simulink model "REGULATORS"  (R2017b)
settings: Solver=VariableStepAuto  StartTime=0.0  StopTime=500  RelTol=1e-3
values from neighbouring files (symbols this model uses):
  A = [dh1dh1 dh1dh2; dh2dh1 dh2dh2]    [SSV_milan.m]    (also in identifikace.m = -0.066; linear_systim.m)
  a_con = 0.075    [SSV_milan.m]
  B = [ dh1du dh1dvt dh1dvo; dh2du dh2dvt dh2dvo ]    [SSV_milan.m]    (also in identifikace.m = -0.0144; linear_systim.m)
  b_con = 0.013    [SSV_milan.m]
  C = [1 0; 0 1]    [SSV_milan.m]    (also in identifikace.m = -0.02; linear_systim.m)
  c_con = 0.02    [SSV_milan.m]
  D = [ 0 0 0; 0 0 0]    [SSV_milan.m]    (also in linear_systim.m)
  d_con = 2.4    [SSV_milan.m]
  h10 = 0.18    [SSV_milan.m]    (also in identifikace_parametru.m = 0.066; linear_systim.m = 0.16)
  h1off = 0.045    [SSV_milan.m]    (also in linear_systim.m = 0.05)
  h20 = 0.08    [SSV_milan.m]    (also in identifikace_parametru.m = 0.175; linear_systim.m = 0.14)
  u0 = 0.4    [SSV_milan.m]    (also in linear_systim.m)
  vO = 1    [SSV_milan.m]    (also in linear_systim.m = 0)
  vT = 1    [SSV_milan.m]    (also in linear_systim.m = 0.5)
libraries: simulink x6
settings Model: Creator=ladislav  LastModifiedBy=ladislav

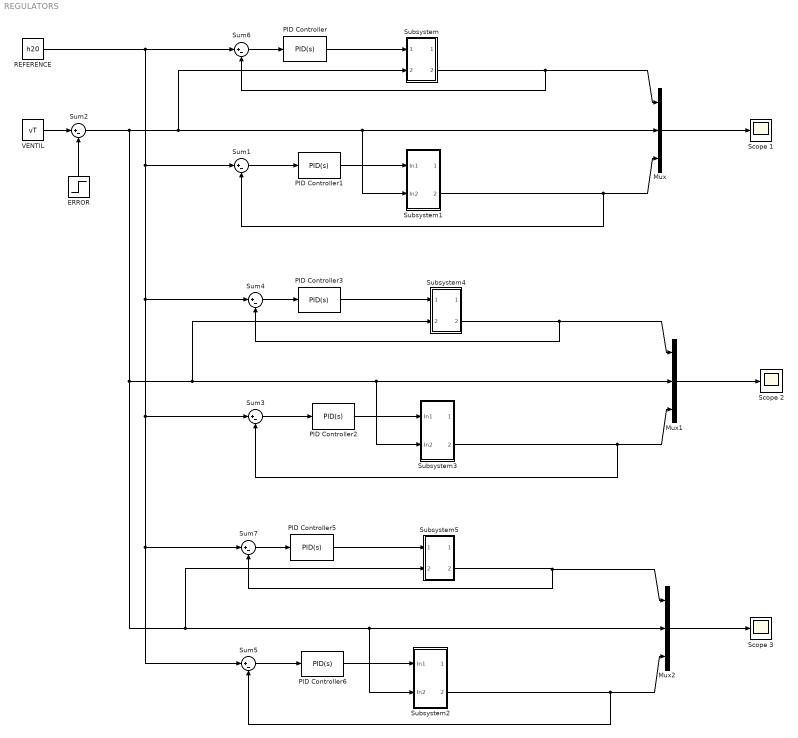
== system REGULATORS ==
  ERROR : Step  Time=200  After=0.2  SampleTime=0  ZeroCross=off
  Mux : Mux  Inputs=3
  Mux1 : Mux  Inputs=3
  Mux2 : Mux  Inputs=3
  PID Controller : simulink/Continuous/PID Controller  Controller=PID  TimeDomain=Continuous-time  SampleTime=-1  IntegratorMethod=Forward Euler  FilterMethod=Forward Euler  Form=Parallel  UseFilter=on  ControllerParametersSource=internal  P=4.4816  I=0.2801  D=0  N=100  InitialConditionSource=internal  InitialConditionForIntegrator=0  InitialConditionForFilter=0  ExternalReset=none  LimitOutput=on  UpperSaturationLimit=1  LowerSaturationLimit=0  LinearizeAsGain=on  AntiWindupMode=none  Kb=1  TrackingMode=off  Kt=1  PParamMin=[]  PParamMax=[]  IParamMin=[]  IParamMax=[]  DParamMin=[]  DParamMax=[]  NParamMin=[]  NParamMax=[]  KbParamMin=[]  KbParamMax=[]  KtParamMin=[]  KtParamMax=[]  POutMin=[]  POutMax=[]  IOutMin=[]  IOutMax=[]  DOutMin=[]  DOutMax=[]  NOutMin=[]  NOutMax=[]  KbOutMin=[]  KbOutMax=[]  KtOutMin=[]  KtOutMax=[]  IntegratorOutMin=[]  IntegratorOutMax=[]  FilterOutMin=[]  FilterOutMax=[]  SumOutMin=[]  SumOutMax=[]  SumI1OutMin=[]  SumI1OutMax=[]  SumI2OutMin=[]  SumI2OutMax=[]  SumI3OutMin=[]  SumI3OutMax=[]  SumDOutMin=[]  SumDOutMax=[]  SaturationOutMin=[]  SaturationOutMax=[]  IntegratorContinuousStateAttributes=''  IntegratorStateMustResolveToSignalObject=off  IntegratorRTWStateStorageClass=Auto  FilterContinuousStateAttributes=''  FilterStateMustResolveToSignalObject=off  FilterRTWStateStorageClass=Auto  DifferentiatorICPrevScaledInput=0  DifferentiatorOutMin=[]  DifferentiatorOutMax=[]  InitialConditionSetting=State (most efficient)  FilterDiffOutCoefMin=[]  FilterDiffOutCoefMax=[]  SumDenOutMin=[]  SumDenOutMax=[]  SumNumOutMin=[]  SumNumOutMax=[]  ReciprocalOutMin=[]  ReciprocalOutMax=[]  DivideOutMin=[]  DivideOutMax=[]  TunerSelectOption=Transfer Function Based (PID Tuner App)
  PID Controller1 : simulink/Continuous/PID Controller  Controller=PID  TimeDomain=Continuous-time  SampleTime=-1  IntegratorMethod=Forward Euler  FilterMethod=Forward Euler  Form=Parallel  UseFilter=on  ControllerParametersSource=internal  P=4.4816  I=0.2801  D=0  N=100  InitialConditionSource=internal  InitialConditionForIntegrator=0  InitialConditionForFilter=0  ExternalReset=none  LimitOutput=on  UpperSaturationLimit=1.0  LowerSaturationLimit=0  LinearizeAsGain=on  AntiWindupMode=none  Kb=1  TrackingMode=off  Kt=1  PParamMin=[]  PParamMax=[]  IParamMin=[]  IParamMax=[]  DParamMin=[]  DParamMax=[]  NParamMin=[]  NParamMax=[]  KbParamMin=[]  KbParamMax=[]  KtParamMin=[]  KtParamMax=[]  POutMin=[]  POutMax=[]  IOutMin=[]  IOutMax=[]  DOutMin=[]  DOutMax=[]  NOutMin=[]  NOutMax=[]  KbOutMin=[]  KbOutMax=[]  KtOutMin=[]  KtOutMax=[]  IntegratorOutMin=[]  IntegratorOutMax=[]  FilterOutMin=[]  FilterOutMax=[]  SumOutMin=[]  SumOutMax=[]  SumI1OutMin=[]  SumI1OutMax=[]  SumI2OutMin=[]  SumI2OutMax=[]  SumI3OutMin=[]  SumI3OutMax=[]  SumDOutMin=[]  SumDOutMax=[]  SaturationOutMin=[]  SaturationOutMax=[]  IntegratorContinuousStateAttributes=''  IntegratorStateMustResolveToSignalObject=off  IntegratorRTWStateStorageClass=Auto  FilterContinuousStateAttributes=''  FilterStateMustResolveToSignalObject=off  FilterRTWStateStorageClass=Auto  DifferentiatorICPrevScaledInput=0  DifferentiatorOutMin=[]  DifferentiatorOutMax=[]  InitialConditionSetting=State (most efficient)  FilterDiffOutCoefMin=[]  FilterDiffOutCoefMax=[]  SumDenOutMin=[]  SumDenOutMax=[]  SumNumOutMin=[]  SumNumOutMax=[]  ReciprocalOutMin=[]  ReciprocalOutMax=[]  DivideOutMin=[]  DivideOutMax=[]  TunerSelectOption=Transfer Function Based (PID Tuner App)
  PID Controller2 : simulink/Continuous/PID Controller  Controller=PID  TimeDomain=Continuous-time  SampleTime=-1  IntegratorMethod=Forward Euler  FilterMethod=Forward Euler  Form=Parallel  UseFilter=on  ControllerParametersSource=internal  P=37.28  I=5.78  D=1.447  N=100  InitialConditionSource=internal  InitialConditionForIntegrator=0  InitialConditionForFilter=0  ExternalReset=none  LimitOutput=on  UpperSaturationLimit=1  LowerSaturationLimit=0  LinearizeAsGain=on  AntiWindupMode=none  Kb=1  TrackingMode=off  Kt=1  PParamMin=[]  PParamMax=[]  IParamMin=[]  IParamMax=[]  DParamMin=[]  DParamMax=[]  NParamMin=[]  NParamMax=[]  KbParamMin=[]  KbParamMax=[]  KtParamMin=[]  KtParamMax=[]  POutMin=[]  POutMax=[]  IOutMin=[]  IOutMax=[]  DOutMin=[]  DOutMax=[]  NOutMin=[]  NOutMax=[]  KbOutMin=[]  KbOutMax=[]  KtOutMin=[]  KtOutMax=[]  IntegratorOutMin=[]  IntegratorOutMax=[]  FilterOutMin=[]  FilterOutMax=[]  SumOutMin=[]  SumOutMax=[]  SumI1OutMin=[]  SumI1OutMax=[]  SumI2OutMin=[]  SumI2OutMax=[]  SumI3OutMin=[]  SumI3OutMax=[]  SumDOutMin=[]  SumDOutMax=[]  SaturationOutMin=[]  SaturationOutMax=[]  IntegratorContinuousStateAttributes=''  IntegratorStateMustResolveToSignalObject=off  IntegratorRTWStateStorageClass=Auto  FilterContinuousStateAttributes=''  FilterStateMustResolveToSignalObject=off  FilterRTWStateStorageClass=Auto  DifferentiatorICPrevScaledInput=0  DifferentiatorOutMin=[]  DifferentiatorOutMax=[]  InitialConditionSetting=State (most efficient)  FilterDiffOutCoefMin=[]  FilterDiffOutCoefMax=[]  SumDenOutMin=[]  SumDenOutMax=[]  SumNumOutMin=[]  SumNumOutMax=[]  ReciprocalOutMin=[]  ReciprocalOutMax=[]  DivideOutMin=[]  DivideOutMax=[]  TunerSelectOption=Transfer Function Based (PID Tuner App)
  PID Controller3 : simulink/Continuous/PID Controller  Controller=PID  TimeDomain=Continuous-time  SampleTime=-1  IntegratorMethod=Forward Euler  FilterMethod=Forward Euler  Form=Parallel  UseFilter=on  ControllerParametersSource=internal  P=37.28  I=5.78  D=1.447  N=100  InitialConditionSource=internal  InitialConditionForIntegrator=0  InitialConditionForFilter=0  ExternalReset=none  LimitOutput=on  UpperSaturationLimit=1  LowerSaturationLimit=0  LinearizeAsGain=on  AntiWindupMode=none  Kb=1  TrackingMode=off  Kt=1  PParamMin=[]  PParamMax=[]  IParamMin=[]  IParamMax=[]  DParamMin=[]  DParamMax=[]  NParamMin=[]  NParamMax=[]  KbParamMin=[]  KbParamMax=[]  KtParamMin=[]  KtParamMax=[]  POutMin=[]  POutMax=[]  IOutMin=[]  IOutMax=[]  DOutMin=[]  DOutMax=[]  NOutMin=[]  NOutMax=[]  KbOutMin=[]  KbOutMax=[]  KtOutMin=[]  KtOutMax=[]  IntegratorOutMin=[]  IntegratorOutMax=[]  FilterOutMin=[]  FilterOutMax=[]  SumOutMin=[]  SumOutMax=[]  SumI1OutMin=[]  SumI1OutMax=[]  SumI2OutMin=[]  SumI2OutMax=[]  SumI3OutMin=[]  SumI3OutMax=[]  SumDOutMin=[]  SumDOutMax=[]  SaturationOutMin=[]  SaturationOutMax=[]  IntegratorContinuousStateAttributes=''  IntegratorStateMustResolveToSignalObject=off  IntegratorRTWStateStorageClass=Auto  FilterContinuousStateAttributes=''  FilterStateMustResolveToSignalObject=off  FilterRTWStateStorageClass=Auto  DifferentiatorICPrevScaledInput=0  DifferentiatorOutMin=[]  DifferentiatorOutMax=[]  InitialConditionSetting=State (most efficient)  FilterDiffOutCoefMin=[]  FilterDiffOutCoefMax=[]  SumDenOutMin=[]  SumDenOutMax=[]  SumNumOutMin=[]  SumNumOutMax=[]  ReciprocalOutMin=[]  ReciprocalOutMax=[]  DivideOutMin=[]  DivideOutMax=[]  TunerSelectOption=Transfer Function Based (PID Tuner App)
  PID Controller5 : simulink/Continuous/PID Controller  Controller=PID  TimeDomain=Continuous-time  SampleTime=-1  IntegratorMethod=Forward Euler  FilterMethod=Forward Euler  Form=Parallel  UseFilter=on  ControllerParametersSource=internal  P=43.1  I=0  D=86.2  N=100  InitialConditionSource=internal  InitialConditionForIntegrator=0  InitialConditionForFilter=0  ExternalReset=none  LimitOutput=on  UpperSaturationLimit=1  LowerSaturationLimit=0  LinearizeAsGain=on  AntiWindupMode=none  Kb=1  TrackingMode=off  Kt=1  PParamMin=[]  PParamMax=[]  IParamMin=[]  IParamMax=[]  DParamMin=[]  DParamMax=[]  NParamMin=[]  NParamMax=[]  KbParamMin=[]  KbParamMax=[]  KtParamMin=[]  KtParamMax=[]  POutMin=[]  POutMax=[]  IOutMin=[]  IOutMax=[]  DOutMin=[]  DOutMax=[]  NOutMin=[]  NOutMax=[]  KbOutMin=[]  KbOutMax=[]  KtOutMin=[]  KtOutMax=[]  IntegratorOutMin=[]  IntegratorOutMax=[]  FilterOutMin=[]  FilterOutMax=[]  SumOutMin=[]  SumOutMax=[]  SumI1OutMin=[]  SumI1OutMax=[]  SumI2OutMin=[]  SumI2OutMax=[]  SumI3OutMin=[]  SumI3OutMax=[]  SumDOutMin=[]  SumDOutMax=[]  SaturationOutMin=[]  SaturationOutMax=[]  IntegratorContinuousStateAttributes=''  IntegratorStateMustResolveToSignalObject=off  IntegratorRTWStateStorageClass=Auto  FilterContinuousStateAttributes=''  FilterStateMustResolveToSignalObject=off  FilterRTWStateStorageClass=Auto  DifferentiatorICPrevScaledInput=0  DifferentiatorOutMin=[]  DifferentiatorOutMax=[]  InitialConditionSetting=State (most efficient)  FilterDiffOutCoefMin=[]  FilterDiffOutCoefMax=[]  SumDenOutMin=[]  SumDenOutMax=[]  SumNumOutMin=[]  SumNumOutMax=[]  ReciprocalOutMin=[]  ReciprocalOutMax=[]  DivideOutMin=[]  DivideOutMax=[]  TunerSelectOption=Transfer Function Based (PID Tuner App)
  PID Controller6 : simulink/Continuous/PID Controller  Controller=PID  TimeDomain=Continuous-time  SampleTime=-1  IntegratorMethod=Forward Euler  FilterMethod=Forward Euler  Form=Parallel  UseFilter=on  ControllerParametersSource=internal  P=43.1  I=0  D=86.2  N=100  InitialConditionSource=internal  InitialConditionForIntegrator=0  InitialConditionForFilter=0  ExternalReset=none  LimitOutput=on  UpperSaturationLimit=1  LowerSaturationLimit=0  LinearizeAsGain=on  AntiWindupMode=none  Kb=1  TrackingMode=off  Kt=1  PParamMin=[]  PParamMax=[]  IParamMin=[]  IParamMax=[]  DParamMin=[]  DParamMax=[]  NParamMin=[]  NParamMax=[]  KbParamMin=[]  KbParamMax=[]  KtParamMin=[]  KtParamMax=[]  POutMin=[]  POutMax=[]  IOutMin=[]  IOutMax=[]  DOutMin=[]  DOutMax=[]  NOutMin=[]  NOutMax=[]  KbOutMin=[]  KbOutMax=[]  KtOutMin=[]  KtOutMax=[]  IntegratorOutMin=[]  IntegratorOutMax=[]  FilterOutMin=[]  FilterOutMax=[]  SumOutMin=[]  SumOutMax=[]  SumI1OutMin=[]  SumI1OutMax=[]  SumI2OutMin=[]  SumI2OutMax=[]  SumI3OutMin=[]  SumI3OutMax=[]  SumDOutMin=[]  SumDOutMax=[]  SaturationOutMin=[]  SaturationOutMax=[]  IntegratorContinuousStateAttributes=''  IntegratorStateMustResolveToSignalObject=off  IntegratorRTWStateStorageClass=Auto  FilterContinuousStateAttributes=''  FilterStateMustResolveToSignalObject=off  FilterRTWStateStorageClass=Auto  DifferentiatorICPrevScaledInput=0  DifferentiatorOutMin=[]  DifferentiatorOutMax=[]  InitialConditionSetting=State (most efficient)  FilterDiffOutCoefMin=[]  FilterDiffOutCoefMax=[]  SumDenOutMin=[]  SumDenOutMax=[]  SumNumOutMin=[]  SumNumOutMax=[]  ReciprocalOutMin=[]  ReciprocalOutMax=[]  DivideOutMin=[]  DivideOutMax=[]  TunerSelectOption=Transfer Function Based (PID Tuner App)
  REFERENCE : Constant  Value=h20
  Scope 1 : Scope
  Scope 2 : Scope
  Scope 3 : Scope
  Subsystem : Subsystem
  Subsystem1 : Subsystem
  Subsystem2 : Subsystem
  Subsystem3 : Subsystem
  Subsystem4 : Subsystem
  Subsystem5 : Subsystem
  Sum{1..7} (7 alike) : Sum  Inputs=|+-
  "VENTIL " : Constant  Value=vT
  wires:
  Sum6/1 -> PID Controller/1
  Subsystem/2(Out2) -> Mux/1, Sum6/2
  PID Controller/1 -> Subsystem/1(In1)
  Sum1/1 -> PID Controller1/1
  PID Controller1/1 -> Subsystem1/1(In1)
  Subsystem1/2(Out2) -> Mux/3, Sum1/2
  Mux/1 -> Scope 1/1
  "VENTIL "/1 -> Sum2/1
  ERROR/1 -> Sum2/2
  PID Controller3/1 -> Subsystem4/1(In1)
  Sum3/1 -> PID Controller2/1
  PID Controller2/1 -> Subsystem3/1(In1)
  Sum4/1 -> PID Controller3/1
  Subsystem3/2(Out2) -> Mux1/3, Sum3/2
  Subsystem4/2(Out2) -> Mux1/1, Sum4/2
  Mux1/1 -> Scope 2/1
  Subsystem5/2(Out2) -> Mux2/1, Sum7/2
  REFERENCE/1 -> Sum7/1, Sum5/1, Sum3/1, Sum4/1, Sum1/1, Sum6/1
  Sum2/1 -> Subsystem5/2(In2), Mux2/2, Subsystem2/2(In2), Subsystem4/2(In2), Mux1/2, Subsystem3/2(In2), Mux/2, Subsystem1/2(In2), Subsystem/2(In2)
  Mux2/1 -> Scope 3/1
  PID Controller6/1 -> Subsystem2/1(In1)
  Sum7/1 -> PID Controller5/1
  Subsystem2/2(Out2) -> Mux2/3, Sum5/2
  PID Controller5/1 -> Subsystem5/1(In1)
  Sum5/1 -> PID Controller6/1

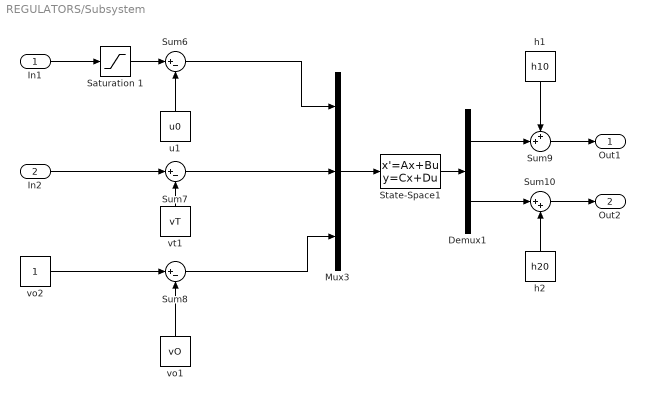
== system REGULATORS/Subsystem ==
  In1 : Inport
  In2 : Inport  Port=2
  Demux1 : Demux  Outputs=2
  Mux3 : Mux  Inputs=3
  Saturation 1 : Saturate  UpperLimit=1
  State-Space1 : StateSpace  A=A  B=B  C=C  D=D  InitialCondition=0
  Sum10 : Sum  Inputs=|++
  Sum6 : Sum  Inputs=|+-
  Sum7 : Sum  Inputs=|+-
  Sum8 : Sum  Inputs=|+-
  Sum9 : Sum  Inputs=++|
  h1 : Constant  Value=h10
  h2 : Constant  Value=h20
  u1 : Constant  Value=u0
  vo1 : Constant  Value=vO
  vo2 : Constant
  vt1 : Constant  Value=vT
  Out1 : Outport
  Out2 : Outport  Port=2
  wires:
  u1/1 -> Sum6/2
  Sum10/1 -> Out2/1
  Sum6/1 -> Mux3/1
  Sum8/1 -> Mux3/3
  h2/1 -> Sum10/2
  vt1/1 -> Sum7/2
  Sum9/1 -> Out1/1
  h1/1 -> Sum9/1
  vo1/1 -> Sum8/2
  In2/1 -> Sum7/1
  Mux3/1 -> State-Space1/1
  Demux1/2 -> Sum10/1
  Sum7/1 -> Mux3/2
  In1/1 -> Saturation 1/1
  State-Space1/1 -> Demux1/1
  Demux1/1 -> Sum9/2
  Saturation 1/1 -> Sum6/1
  vo2/1 -> Sum8/1

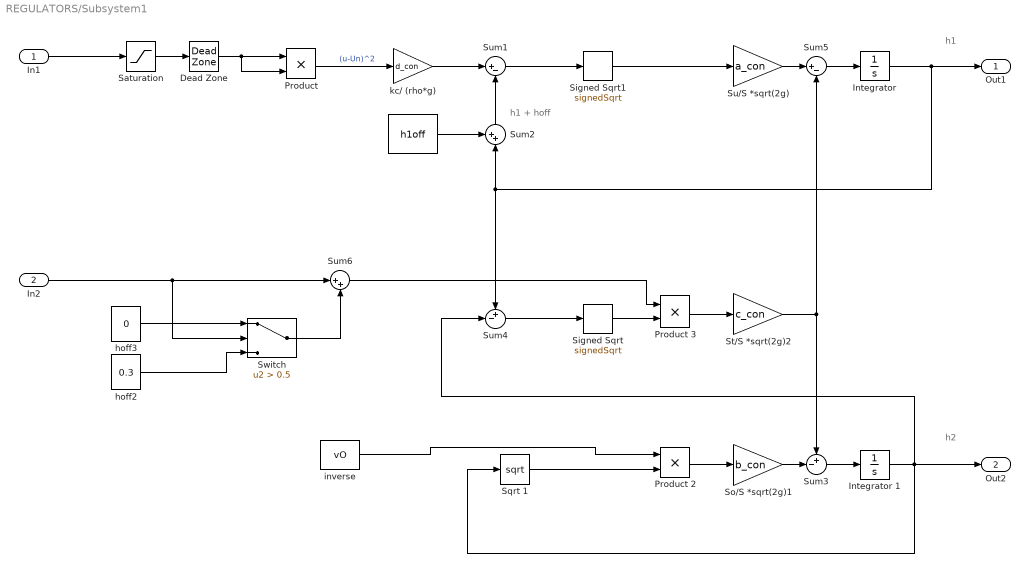
== system REGULATORS/Subsystem1 ==
  note: h1
  note: h1 + hoff
  note: h2
  In1 : Inport
  In2 : Inport  Port=2
  " " : Constant  Value=h1off
  " hoff2" : Constant  Value=0.3
  " hoff3" : Constant  Value=0
  " inverse" : Constant  Value=vO
  "Dead Zone " : DeadZone  LowerValue=0  UpperValue=0.05  SaturateOnIntegerOverflow=on
  "Integrator " : Integrator  InitialCondition=-0.045  LimitOutput=on  UpperSaturationLimit=0.71  LowerSaturationLimit=-0.045
  Integrator 1 : Integrator  LimitOutput=on  UpperSaturationLimit=0.71  LowerSaturationLimit=0
  "Product " : Product
  Product 2 : Product
  Product 3 : Product
  "Saturation " : Saturate  UpperLimit=1
  Signed Sqrt : Sqrt  Operator=signedSqrt  SaturateOnIntegerOverflow=on
  Signed Sqrt1 : Sqrt  Operator=signedSqrt  SaturateOnIntegerOverflow=on
  So/S *sqrt(2g)1 : Gain  Gain=b_con
  Sqrt 1 : Sqrt  SaturateOnIntegerOverflow=on
  St/S *sqrt(2g)2 : Gain  Gain=c_con
  Su/S *sqrt(2g) : Gain  Gain=a_con
  Sum1 : Sum  Inputs=|+-
  Sum2 : Sum  Inputs=++|
  Sum3 : Sum  Inputs=+-|
  Sum4 : Sum  Inputs=+-|
  Sum5 : Sum  Inputs=|+-
  Sum6 : Sum  Inputs=|++
  Switch : Switch  Criteria=u2 > Threshold  Threshold=0.5
  kc/ (rho*g) : Gain  Gain=d_con
  Out1 : Outport
  Out2 : Outport  Port=2
  wires:
  In1/1 -> "Saturation "/1
  Sum6/1 -> Product 3/1
  " hoff2"/1 -> Switch/3
  "Saturation "/1 -> "Dead Zone "/1
  "Integrator "/1 -> Out1/1, Sum2/2, Sum4/1
  Sqrt 1/1 -> Product 2/2
  "Dead Zone "/1 -> "Product "/2, "Product "/1
  " "/1 -> Sum2/1
  kc/ (rho*g)/1 -> Sum1/1
  Sum5/1 -> "Integrator "/1
  Sum2/1 -> Sum1/2
  Integrator 1/1 -> Sum4/2, Out2/1, Sqrt 1/1
  In2/1 -> Switch/2, Sum6/1
  So/S *sqrt(2g)1/1 -> Sum3/2
  Sum3/1 -> Integrator 1/1
  Product 3/1 -> St/S *sqrt(2g)2/1
  "Product "/1 -> kc/ (rho*g)/1  "(u-Un)^2"
  Product 2/1 -> So/S *sqrt(2g)1/1
  " inverse"/1 -> Product 2/1
  St/S *sqrt(2g)2/1 -> Sum5/2, Sum3/1
  " hoff3"/1 -> Switch/1
  Switch/1 -> Sum6/2
  Sum4/1 -> Signed Sqrt/1
  Signed Sqrt/1 -> Product 3/2
  Sum1/1 -> Signed Sqrt1/1
  Signed Sqrt1/1 -> Su/S *sqrt(2g)/1
  Su/S *sqrt(2g)/1 -> Sum5/1

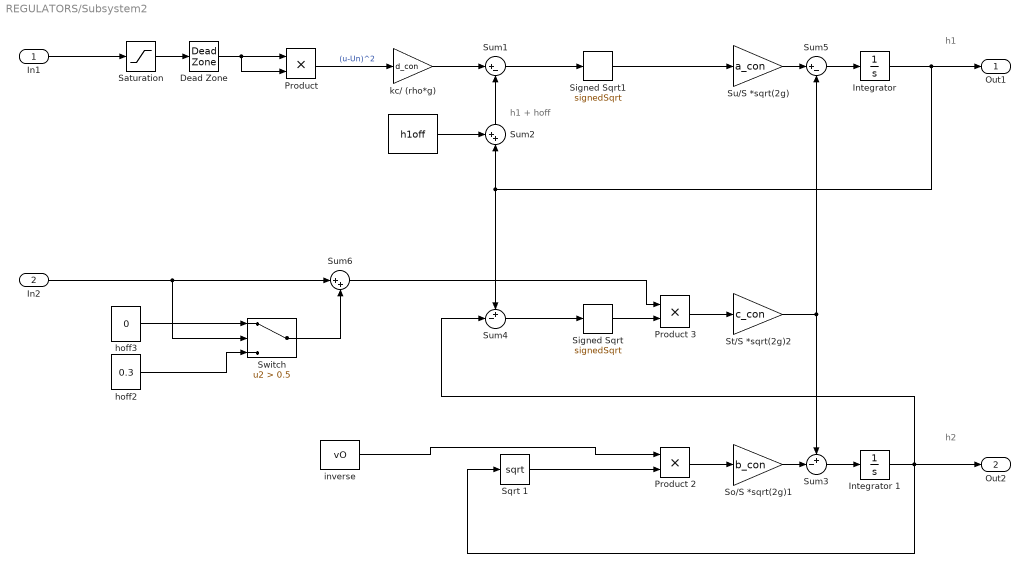
== system REGULATORS/Subsystem2 ==
  note: h1
  note: h1 + hoff
  note: h2
  In1 : Inport
  In2 : Inport  Port=2
  " " : Constant  Value=h1off
  " hoff2" : Constant  Value=0.3
  " hoff3" : Constant  Value=0
  " inverse" : Constant  Value=vO
  "Dead Zone " : DeadZone  LowerValue=0  UpperValue=0.05  SaturateOnIntegerOverflow=on
  "Integrator " : Integrator  InitialCondition=-0.045  LimitOutput=on  UpperSaturationLimit=0.71  LowerSaturationLimit=-0.045
  Integrator 1 : Integrator  LimitOutput=on  UpperSaturationLimit=0.71  LowerSaturationLimit=0
  "Product " : Product
  Product 2 : Product
  Product 3 : Product
  "Saturation " : Saturate  UpperLimit=1
  Signed Sqrt : Sqrt  Operator=signedSqrt  SaturateOnIntegerOverflow=on
  Signed Sqrt1 : Sqrt  Operator=signedSqrt  SaturateOnIntegerOverflow=on
  So/S *sqrt(2g)1 : Gain  Gain=b_con
  Sqrt 1 : Sqrt  SaturateOnIntegerOverflow=on
  St/S *sqrt(2g)2 : Gain  Gain=c_con
  Su/S *sqrt(2g) : Gain  Gain=a_con
  Sum1 : Sum  Inputs=|+-
  Sum2 : Sum  Inputs=++|
  Sum3 : Sum  Inputs=+-|
  Sum4 : Sum  Inputs=+-|
  Sum5 : Sum  Inputs=|+-
  Sum6 : Sum  Inputs=|++
  Switch : Switch  Criteria=u2 > Threshold  Threshold=0.5
  kc/ (rho*g) : Gain  Gain=d_con
  Out1 : Outport
  Out2 : Outport  Port=2
  wires:
  In1/1 -> "Saturation "/1
  Sum6/1 -> Product 3/1
  " hoff2"/1 -> Switch/3
  "Saturation "/1 -> "Dead Zone "/1
  "Integrator "/1 -> Out1/1, Sum2/2, Sum4/1
  Sqrt 1/1 -> Product 2/2
  "Dead Zone "/1 -> "Product "/2, "Product "/1
  " "/1 -> Sum2/1
  kc/ (rho*g)/1 -> Sum1/1
  Sum5/1 -> "Integrator "/1
  Sum2/1 -> Sum1/2
  Integrator 1/1 -> Sum4/2, Out2/1, Sqrt 1/1
  In2/1 -> Switch/2, Sum6/1
  So/S *sqrt(2g)1/1 -> Sum3/2
  Sum3/1 -> Integrator 1/1
  Product 3/1 -> St/S *sqrt(2g)2/1
  "Product "/1 -> kc/ (rho*g)/1  "(u-Un)^2"
  Product 2/1 -> So/S *sqrt(2g)1/1
  " inverse"/1 -> Product 2/1
  St/S *sqrt(2g)2/1 -> Sum5/2, Sum3/1
  " hoff3"/1 -> Switch/1
  Switch/1 -> Sum6/2
  Sum4/1 -> Signed Sqrt/1
  Signed Sqrt/1 -> Product 3/2
  Sum1/1 -> Signed Sqrt1/1
  Signed Sqrt1/1 -> Su/S *sqrt(2g)/1
  Su/S *sqrt(2g)/1 -> Sum5/1

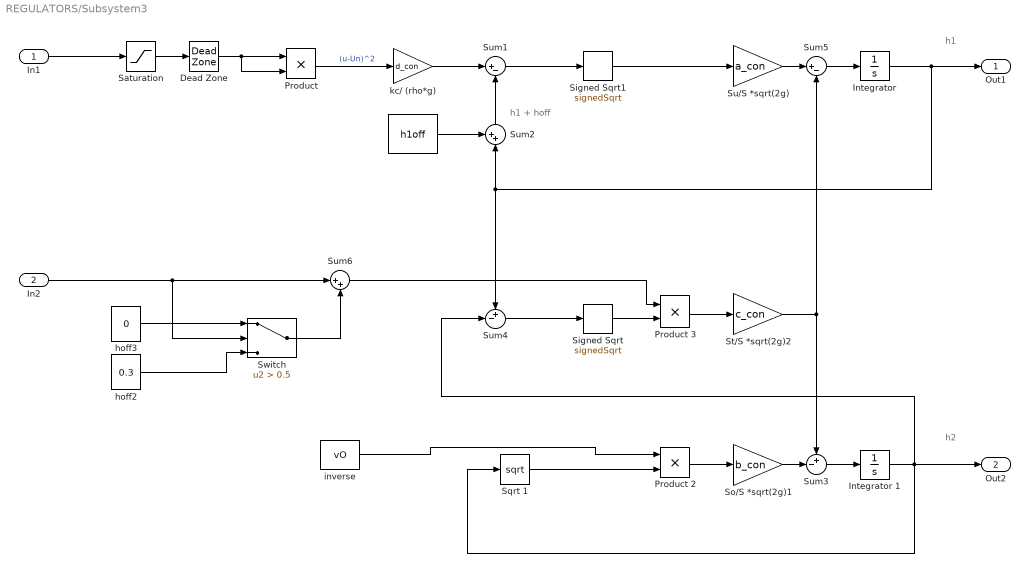
== system REGULATORS/Subsystem3 ==
  note: h1
  note: h1 + hoff
  note: h2
  In1 : Inport
  In2 : Inport  Port=2
  " " : Constant  Value=h1off
  " hoff2" : Constant  Value=0.3
  " hoff3" : Constant  Value=0
  " inverse" : Constant  Value=vO
  "Dead Zone " : DeadZone  LowerValue=0  UpperValue=0.05  SaturateOnIntegerOverflow=on
  "Integrator " : Integrator  InitialCondition=-0.045  LimitOutput=on  UpperSaturationLimit=0.71  LowerSaturationLimit=-0.045
  Integrator 1 : Integrator  LimitOutput=on  UpperSaturationLimit=0.71  LowerSaturationLimit=0
  "Product " : Product
  Product 2 : Product
  Product 3 : Product
  "Saturation " : Saturate  UpperLimit=1
  Signed Sqrt : Sqrt  Operator=signedSqrt  SaturateOnIntegerOverflow=on
  Signed Sqrt1 : Sqrt  Operator=signedSqrt  SaturateOnIntegerOverflow=on
  So/S *sqrt(2g)1 : Gain  Gain=b_con
  Sqrt 1 : Sqrt  SaturateOnIntegerOverflow=on
  St/S *sqrt(2g)2 : Gain  Gain=c_con
  Su/S *sqrt(2g) : Gain  Gain=a_con
  Sum1 : Sum  Inputs=|+-
  Sum2 : Sum  Inputs=++|
  Sum3 : Sum  Inputs=+-|
  Sum4 : Sum  Inputs=+-|
  Sum5 : Sum  Inputs=|+-
  Sum6 : Sum  Inputs=|++
  Switch : Switch  Criteria=u2 > Threshold  Threshold=0.5
  kc/ (rho*g) : Gain  Gain=d_con
  Out1 : Outport
  Out2 : Outport  Port=2
  wires:
  In1/1 -> "Saturation "/1
  Sum6/1 -> Product 3/1
  " hoff2"/1 -> Switch/3
  "Saturation "/1 -> "Dead Zone "/1
  "Integrator "/1 -> Out1/1, Sum2/2, Sum4/1
  Sqrt 1/1 -> Product 2/2
  "Dead Zone "/1 -> "Product "/2, "Product "/1
  " "/1 -> Sum2/1
  kc/ (rho*g)/1 -> Sum1/1
  Sum5/1 -> "Integrator "/1
  Sum2/1 -> Sum1/2
  Integrator 1/1 -> Sum4/2, Out2/1, Sqrt 1/1
  In2/1 -> Switch/2, Sum6/1
  So/S *sqrt(2g)1/1 -> Sum3/2
  Sum3/1 -> Integrator 1/1
  Product 3/1 -> St/S *sqrt(2g)2/1
  "Product "/1 -> kc/ (rho*g)/1  "(u-Un)^2"
  Product 2/1 -> So/S *sqrt(2g)1/1
  " inverse"/1 -> Product 2/1
  St/S *sqrt(2g)2/1 -> Sum5/2, Sum3/1
  " hoff3"/1 -> Switch/1
  Switch/1 -> Sum6/2
  Sum4/1 -> Signed Sqrt/1
  Signed Sqrt/1 -> Product 3/2
  Sum1/1 -> Signed Sqrt1/1
  Signed Sqrt1/1 -> Su/S *sqrt(2g)/1
  Su/S *sqrt(2g)/1 -> Sum5/1

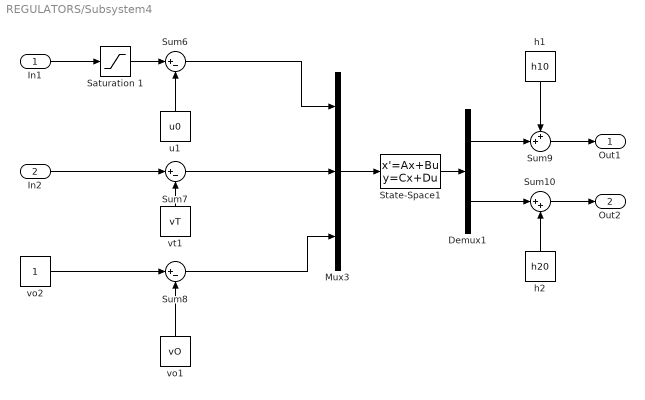
== system REGULATORS/Subsystem4 ==
  In1 : Inport
  In2 : Inport  Port=2
  Demux1 : Demux  Outputs=2
  Mux3 : Mux  Inputs=3
  Saturation 1 : Saturate  UpperLimit=1
  State-Space1 : StateSpace  A=A  B=B  C=C  D=D  InitialCondition=0
  Sum10 : Sum  Inputs=|++
  Sum6 : Sum  Inputs=|+-
  Sum7 : Sum  Inputs=|+-
  Sum8 : Sum  Inputs=|+-
  Sum9 : Sum  Inputs=++|
  h1 : Constant  Value=h10
  h2 : Constant  Value=h20
  u1 : Constant  Value=u0
  vo1 : Constant  Value=vO
  vo2 : Constant
  vt1 : Constant  Value=vT
  Out1 : Outport
  Out2 : Outport  Port=2
  wires:
  u1/1 -> Sum6/2
  Sum10/1 -> Out2/1
  Sum6/1 -> Mux3/1
  Sum8/1 -> Mux3/3
  h2/1 -> Sum10/2
  vt1/1 -> Sum7/2
  Sum9/1 -> Out1/1
  h1/1 -> Sum9/1
  vo1/1 -> Sum8/2
  In2/1 -> Sum7/1
  Mux3/1 -> State-Space1/1
  Demux1/2 -> Sum10/1
  Sum7/1 -> Mux3/2
  In1/1 -> Saturation 1/1
  State-Space1/1 -> Demux1/1
  Demux1/1 -> Sum9/2
  Saturation 1/1 -> Sum6/1
  vo2/1 -> Sum8/1

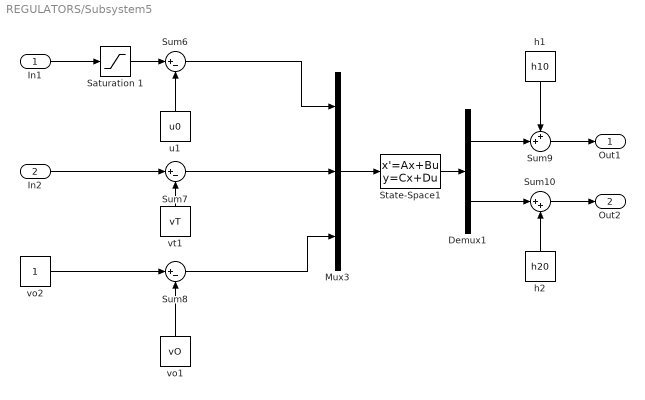
== system REGULATORS/Subsystem5 ==
  In1 : Inport
  In2 : Inport  Port=2
  Demux1 : Demux  Outputs=2
  Mux3 : Mux  Inputs=3
  Saturation 1 : Saturate  UpperLimit=1
  State-Space1 : StateSpace  A=A  B=B  C=C  D=D  InitialCondition=0
  Sum10 : Sum  Inputs=|++
  Sum6 : Sum  Inputs=|+-
  Sum7 : Sum  Inputs=|+-
  Sum8 : Sum  Inputs=|+-
  Sum9 : Sum  Inputs=++|
  h1 : Constant  Value=h10
  h2 : Constant  Value=h20
  u1 : Constant  Value=u0
  vo1 : Constant  Value=vO
  vo2 : Constant
  vt1 : Constant  Value=vT
  Out1 : Outport
  Out2 : Outport  Port=2
  wires:
  u1/1 -> Sum6/2
  Sum10/1 -> Out2/1
  Sum6/1 -> Mux3/1
  Sum8/1 -> Mux3/3
  h2/1 -> Sum10/2
  vt1/1 -> Sum7/2
  Sum9/1 -> Out1/1
  h1/1 -> Sum9/1
  vo1/1 -> Sum8/2
  In2/1 -> Sum7/1
  Mux3/1 -> State-Space1/1
  Demux1/2 -> Sum10/1
  Sum7/1 -> Mux3/2
  In1/1 -> Saturation 1/1
  State-Space1/1 -> Demux1/1
  Demux1/1 -> Sum9/2
  Saturation 1/1 -> Sum6/1
  vo2/1 -> Sum8/1
